simulink model "Relay_Signal_Template"  (R2021a)
settings: Solver=VariableStepAuto  StartTime=0.0  StopTime=10.0  RelTol=1e-3
settings Model: Creator=Intuito_PC  LastModifiedBy=Intuito_PC

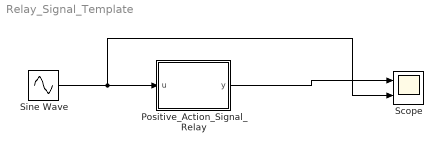
== system Relay_Signal_Template ==
  Positive_Action_Signal_Relay : MATLAB Function  TreatAsAtomicUnit=on
  Scope : Scope  NumInputPorts=2
  Sine Wave : Sin  Amplitude=4  SampleTime=0
  wires:
  Sine Wave/1 -> Scope/2, Positive_Action_Signal_Relay/1(u)
  Positive_Action_Signal_Relay/1(y) -> Scope/1

== matlab function Relay_Signal_Template/Positive_Action_Signal_Relay ==
  data: u input; y output
function y = fcn(u)
% Define limit
limit = 3.0;
if u > limit
    y = 1;
else
    y = 0;
end
end
